simulink model "SpatialKineticsOffline"  (R2013a)
settings: Solver=ode4  StartTime=0.0  StopTime=tf  FixedStep=.001  RelTol=1e-3
PreLoadFcn:
  | load DarkLowerCoeffs
  | load DarkMiddleCoeffs
  | load DarkUpperCoeffs
  | load breaks
values from neighbouring files (symbols this model uses):
  alpha = [ -2.61*pcm -0.53*pcm ]    [SpatialKineticsOpenSourceMain.m]
  breaks = DarkLowerBreaks    [SpatialKineticsOpenSourceMain.m]
  BRIO = 4.266e7    (= 42660000)    [SpatialKineticsOpenSourceMain.m]
  cpc = 2414    [SpatialKineticsOpenSourceMain.m]
  cpp = 2414    [SpatialKineticsOpenSourceMain.m]
  DarkLowerCoeffs = ppDarkLower.coefs    [SpatialKineticsOpenSourceMain.m]
  DarkMiddleCoeffs = ppDarkMiddle.coefs    [SpatialKineticsOpenSourceMain.m]
  DarkRodWorthInserted = -5*Beta    (= -0.00815)    [SpatialKineticsOpenSourceMain.m]
  DarkUpperCoeffs = ppDarkUpper.coefs    [SpatialKineticsOpenSourceMain.m]
  downcomerTimeConstant = 5    [SpatialKineticsOpenSourceMain.m]
  downIO = 216.6*ones(1,3)    [SpatialKineticsOpenSourceMain.m]
  Kc1 = 1/(rho_secondary*V_secondary)    (= 0.00032726218348)    [SpatialKineticsOpenSourceMain.m]
  Kc2 = (h_secondary*A)/(cps*rho_secondary*V_secondary)    (= 1.23242359038)    [SpatialKineticsOpenSourceMain.m]
  Kh1 = 1/(rho_primary*V_primary)    (= 0.000447917898441)    [SpatialKineticsOpenSourceMain.m]
  Kh2 = (h_primary*A)/(cpp*rho_primary*V_primary)    (= 1.29038206968)    [SpatialKineticsOpenSourceMain.m]
  Kw1 = h_primary    (= 23800)    [SpatialKineticsOpenSourceMain.m]
  Kw2 = h_secondary    (= 24500)    [SpatialKineticsOpenSourceMain.m]
  Kw3 = A/(rho_tube*cpw*V_tube)    (= 0.000122049789882)    [SpatialKineticsOpenSourceMain.m]
  PHX_IO = [649.8 637.9 643.7]    [SpatialKineticsOpenSourceMain.m]
  PHX_PI_IO = 271.8    [SpatialKineticsOpenSourceMain.m]
  rate_pct = rate/100    [SpatialKineticsOfflineMain.m]
  rcp_activatetime = 20    [SpatialKineticsOpenSourceMain.m]
  rcpt = 0.1    [SpatialKineticsOpenSourceMain.m]
  reactor_PI_IO = 0.8574    [SpatialKineticsOpenSourceMain.m]
  SVIO = zeros(1,17)    [SpatialKineticsOpenSourceMain.m]
  Ts = 0.001    [SpatialKineticsOpenSourceMain.m]
  xfc0 = -Atemp\btemp*u0    [SpatialKineticsOpenSourceMain.m]
  zone1_IO = [1.041 0.01764 0.04848]    [SpatialKineticsOpenSourceMain.m]
  zone1_thermal_IO = [1044 658.3]    [SpatialKineticsOpenSourceMain.m]
  zone2_IO = [1.098 0.0186 0.05114]    [SpatialKineticsOpenSourceMain.m]
  zone2_thermal_IO = [1083 675.9]    [SpatialKineticsOpenSourceMain.m]
  zone3_IO = [0.9147 0.01549 0.04259]    [SpatialKineticsOpenSourceMain.m]
  zone3_thermal_IO = [1031 692.5]    [SpatialKineticsOpenSourceMain.m]
libraries: simulink x36
(part 1 of 5)
settings Model: BufferReuse=off  Creator=LabUser  LastModifiedBy=LabUser
settings DataIOCC: LimitDataPoints=off
settings OptimizationCC: BlockReduction=off  OptimizeBlockIOStorage=off  BufferReuse=off  ExpressionFolding=off  LocalBlockOutputs=off
settings HardwareCC: ProdIntDivRoundTo=Zero  ProdEndianess=LittleEndian  ProdHWDeviceType=Generic->32-bit x86 compatible
settings RTWCC: SystemTargetFile=xpctarget.tlc  TemplateMakefile=xpc_default_tmf  Description=xPC Target  ProcessScript=xpctarget_make_rtw_hook  RTWCompilerOptimization=On
settings TargetCC: CodeReplacementLibrary=XPC_BLAS  IsPILTarget=off  ParMdlRefBuildCompliant=on  ConcurrentExecutionCompliant=on  MatFileLogging=on  EnableShiftOperators=on  MATLABClassNameForMDSCustomization=xpcAperiodicCustomization

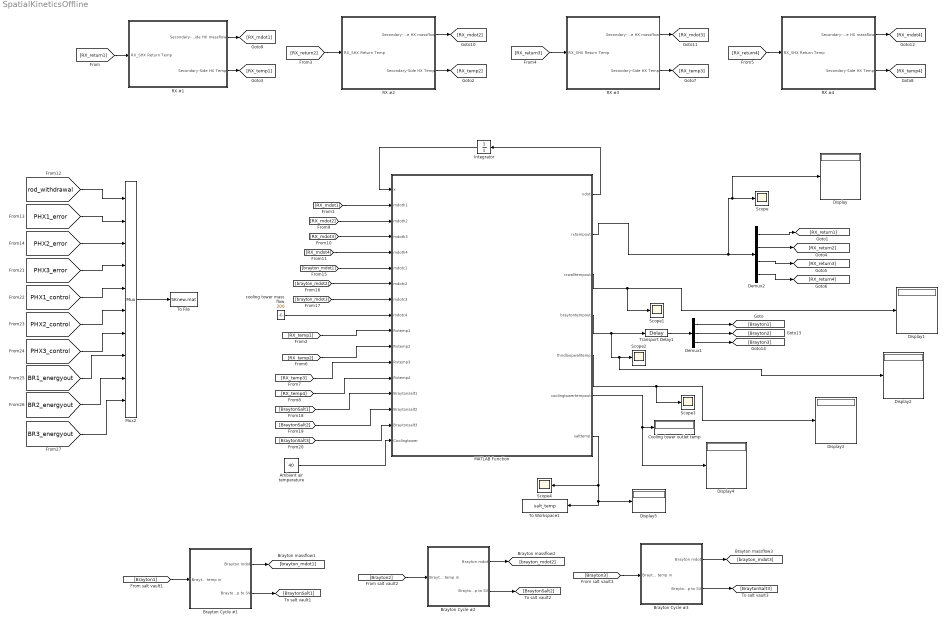
== system SpatialKineticsOffline ==
  Ambient air temperature : Constant  Value=40
  Brayton Cycle #1 : Subsystem
  Brayton Cycle #2 : Subsystem
  Brayton Cycle #3 : Subsystem
  Cooling tower outlet temp : Display
  Demux1 : Demux  Outputs=3
  Demux2 : Demux
  Display{,1..5} (6 alike) : Display
  Integrator : Integrator  InitialCondition=SVIO
  MATLAB Function : MATLAB Function  TreatAsAtomicUnit=on
  Mux2 : Mux  Inputs=10
  RX #1 : Subsystem
  RX #2 : Subsystem
  RX #3 : Subsystem
  RX #4 : Subsystem
  Scope{,1..4} (5 alike) : Scope
      Scope settings: TimeRange=100  YMin=0  YMax=85
      Scope1 settings: TimeRange=100  YMin=0  YMax=85  SaveName=ScopeData3
      Scope2 settings: TimeRange=100  YMin=0  YMax=85  SaveName=ScopeData4
      Scope3 settings: TimeRange=100  YMin=0  YMax=85  SaveName=ScopeData5
      Scope4 settings: TimeRange=100  YMin=0  YMax=85  SaveName=ScopeData6
  To File : ToFile  Filename=SKnew.mat  MatrixName=SKnew
  To Workspace1 : ToWorkspace  VariableName=salt_temp  SampleTime=-1
  Transport Delay1 : TransportDelay
  cooling tower mass flow : Constant  Value=200
  wires:
  RX #1/2(Secondary-Side HX Temp) -> [RX_temp1]
  RX #2/2(Secondary-Side HX Temp) -> [RX_temp2]
  RX #3/2(Secondary-Side HX Temp) -> [RX_temp3]
  RX #4/2(Secondary-Side HX Temp) -> [RX_temp4]
  RX #1/1(Secondary-Side HX massflow) -> [RX_mdot1]
  RX #2/1(Secondary-Side HX massflow) -> [RX_mdot2]
  RX #3/1(Secondary-Side HX massflow) -> [RX_mdot3]
  RX #4/1(Secondary-Side HX massflow) -> [RX_mdot4]
  [RX_return1] -> RX #1/1(RX_SHX Return Temp)
  [RX_return2] -> RX #2/1(RX_SHX Return Temp)
  [RX_return3] -> RX #3/1(RX_SHX Return Temp)
  [RX_return4] -> RX #4/1(RX_SHX Return Temp)
  [Brayton3] -> Brayton Cycle #3/1(Brayton temp in)
  Brayton Cycle #3/1(Brayton mdot) -> [brayton_mdot3]
  Brayton Cycle #3/2(Brayton Temp to SV) -> [BraytonSalt3]
  [Brayton1] -> Brayton Cycle #1/1(Brayton temp in)
  Brayton Cycle #1/1(Brayton mdot) -> [brayton_mdot1]
  Brayton Cycle #1/2(Brayton Temp to SV) -> [BraytonSalt1]
  [Brayton2] -> Brayton Cycle #2/1(Brayton temp in)
  Brayton Cycle #2/1(Brayton mdot) -> [brayton_mdot2]
  Brayton Cycle #2/2(Brayton Temp to SV) -> [BraytonSalt2]
  [rod_withdrawal] -> Mux2/1
  [PHX1_error] -> Mux2/2
  [PHX2_error] -> Mux2/3
  [PHX3_error] -> Mux2/4
  [PHX1_control] -> Mux2/5
  [PHX2_control] -> Mux2/6
  [PHX3_control] -> Mux2/7
  [BR1_energyout] -> Mux2/8
  [BR2_energyout] -> Mux2/9
  [BR3_energyout] -> Mux2/10
  Mux2/1 -> To File/1
  MATLAB Function/1(xdot) -> Integrator/1
  Integrator/1 -> MATLAB Function/1(x)
  MATLAB Function/2(rxtempout) -> Display/1, Scope/1, Demux2/1
  MATLAB Function/6(coolingtowertempout) -> Cooling tower outlet temp/1, Display4/1
  Transport Delay1/1 -> Demux1/1
  Demux1/1 -> [Brayton1]
  Demux1/2 -> [Brayton2]
  cooling tower mass flow/1 -> MATLAB Function/9(mdotc4)
  [brayton_mdot3] -> MATLAB Function/8(mdotc3)
  [brayton_mdot2] -> MATLAB Function/7(mdotc2)
  [brayton_mdot1] -> MATLAB Function/6(mdotc1)
  [RX_mdot4] -> MATLAB Function/5(mdoth4)
  [RX_mdot3] -> MATLAB Function/4(mdoth3)
  [RX_mdot2] -> MATLAB Function/3(mdoth2)
  [RX_mdot1] -> MATLAB Function/2(mdoth1)
  Demux2/2 -> [RX_return2]
  Demux2/3 -> [RX_return3]
  Demux2/4 -> [RX_return4]
  Demux2/1 -> [RX_return1]
  Demux1/3 -> [Brayton3]
  MATLAB Function/4(braytontempout) -> Display2/1, Scope2/1, Transport Delay1/1
  [RX_temp1] -> MATLAB Function/10(Rxtemp1)
  [RX_temp2] -> MATLAB Function/11(Rxtemp2)
  [RX_temp3] -> MATLAB Function/12(Rxtemp3)
  [RX_temp4] -> MATLAB Function/13(Rxtemp4)
  [BraytonSalt1] -> MATLAB Function/14(Braytonsalt1)
  [BraytonSalt2] -> MATLAB Function/15(Braytonsalt2)
  [BraytonSalt3] -> MATLAB Function/16(Braytonsalt3)
  Ambient air temperature/1 -> MATLAB Function/17(Coolingtower)
  MATLAB Function/3(rxwalltempout) -> Scope1/1, Display1/1
  MATLAB Function/5(thirdloopwalltemp) -> Scope3/1, Display3/1
  MATLAB Function/7(salttemp) -> To Workspace1/1, Display5/1, Scope4/1

== system SpatialKineticsOffline/Brayton Cycle #1 ==
  Brayton temp in : Inport
  Brayton Cycle Parameters : FromWorkspace  VariableName=[0,eta_C,eta_T,r,cpCO2Turbine,cpCO2Compressor,rhoCO2,tau_t]  SampleTime=0
  Compressor Inlet Temp : Constant  Value=10
  Display : Display
  Electricity Extraction : Display
  Generator Efficiency : Gain  Gain=0.60
  Integrator : Integrator  InitialCondition=BRIO
  MATLAB Function : MATLAB Function  TreatAsAtomicUnit=on
  Mux4 : Mux  Inputs=2
  Terminator : Terminator
  Watts to MW : Gain  Gain=1/1000000
  kg/s : Constant  Value=500
  Brayton mdot : Outport
  Brayton Temp to SV : Outport  Port=2
  tag scope: BR1_energyout=global
  wires:
  Brayton Cycle Parameters/1 -> MATLAB Function/4(constants)
  Integrator/1 -> MATLAB Function/5(x), Display/1
  kg/s/1 -> MATLAB Function/3(mdot), Brayton mdot/1
  MATLAB Function/4(xdot) -> Integrator/1
  Brayton temp in/1 -> MATLAB Function/2(Tturb_in)
  Compressor Inlet Temp/1 -> MATLAB Function/1(Tcomp_in)
  Generator Efficiency/1 -> [BR1_energyout], Electricity Extraction/1
  Mux4/1 -> Terminator/1
  MATLAB Function/3(Tcomp_out) -> Brayton Temp to SV/1, Mux4/2
  MATLAB Function/1(y) -> Watts to MW/1
  Watts to MW/1 -> Generator Efficiency/1
  MATLAB Function/2(Tturb_out) -> Mux4/1

== system SpatialKineticsOffline/Brayton Cycle #2 ==
  Brayton temp in : Inport
  Brayton Cycle Parameters2 : FromWorkspace  VariableName=[0,eta_C,eta_T,r,cpCO2Turbine,cpCO2Compressor,rhoCO2,tau_t]  SampleTime=0
  Compressor Inlet Temp2 : Constant  Value=10
  Display : Display
  Electricity Extraction2 : Display
  Generator Efficiency2 : Gain  Gain=0.60
  Integrator3 : Integrator  InitialCondition=BRIO
  MATLAB Function4 : MATLAB Function  TreatAsAtomicUnit=on
  Mechanical Power Extraction2 : Display
  Mux4 : Mux  Inputs=2
  Terminator : Terminator
  Watts to MW3 : Gain  Gain=1/1000000
  kg/s2 : Constant  Value=500
  Brayton mdot : Outport
  Brayton Temp to SV : Outport  Port=2
  tag scope: BR2_energyout=global
  wires:
  Brayton Cycle Parameters2/1 -> MATLAB Function4/4(constants)
  Integrator3/1 -> MATLAB Function4/5(x), Display/1
  kg/s2/1 -> MATLAB Function4/3(mdot), Brayton mdot/1
  MATLAB Function4/4(xdot) -> Integrator3/1
  Brayton temp in/1 -> MATLAB Function4/2(Tturb_in)
  Compressor Inlet Temp2/1 -> MATLAB Function4/1(Tcomp_in)
  Generator Efficiency2/1 -> [BR2_energyout], Electricity Extraction2/1
  Mux4/1 -> Terminator/1
  MATLAB Function4/3(Tcomp_out) -> Brayton Temp to SV/1, Mux4/2
  MATLAB Function4/1(y) -> Watts to MW3/1
  Watts to MW3/1 -> Generator Efficiency2/1, Mechanical Power Extraction2/1
  MATLAB Function4/2(Tturb_out) -> Mux4/1

== system SpatialKineticsOffline/Brayton Cycle #3 ==
  Brayton temp in : Inport
  Brayton Cycle Parameters2 : FromWorkspace  VariableName=[0,eta_C,eta_T,r,cpCO2Turbine,cpCO2Compressor,rhoCO2,tau_t]  SampleTime=0
  Compressor Inlet Temp2 : Constant  Value=10
  Display : Display
  Electricity Extraction2 : Display
  Generator Efficiency2 : Gain  Gain=0.60
  Integrator3 : Integrator  InitialCondition=BRIO
  MATLAB Function4 : MATLAB Function  TreatAsAtomicUnit=on
  Mechanical Power Extraction2 : Display
  Mux4 : Mux  Inputs=2
  Terminator : Terminator
  Watts to MW3 : Gain  Gain=1/1000000
  kg/s2 : Constant  Value=500
  Brayton mdot : Outport
  Brayton Temp to SV : Outport  Port=2
  tag scope: BR3_energyout=global
  wires:
  Brayton Cycle Parameters2/1 -> MATLAB Function4/4(constants)
  Integrator3/1 -> Display/1, MATLAB Function4/5(x)
  kg/s2/1 -> MATLAB Function4/3(mdot), Brayton mdot/1
  MATLAB Function4/4(xdot) -> Integrator3/1
  Brayton temp in/1 -> MATLAB Function4/2(Tturb_in)
  Compressor Inlet Temp2/1 -> MATLAB Function4/1(Tcomp_in)
  Generator Efficiency2/1 -> [BR3_energyout], Electricity Extraction2/1
  Mux4/1 -> Terminator/1
  MATLAB Function4/3(Tcomp_out) -> Brayton Temp to SV/1, Mux4/2
  MATLAB Function4/1(y) -> Watts to MW3/1
  Watts to MW3/1 -> Generator Efficiency2/1, Mechanical Power Extraction2/1
  MATLAB Function4/2(Tturb_out) -> Mux4/1

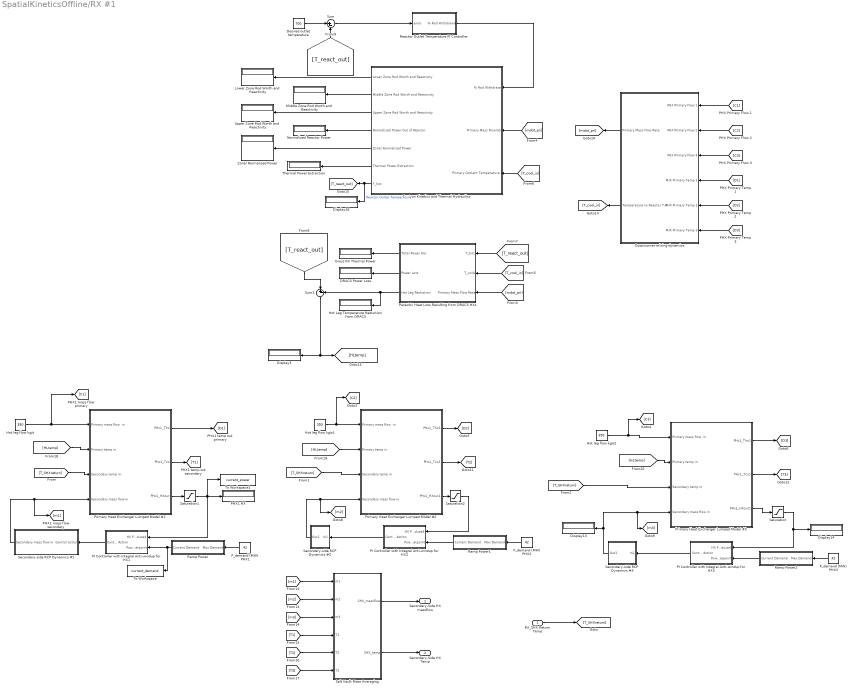
== system SpatialKineticsOffline/RX #1 ==
  RX_SHX Return Temp : Inport
  DRACS Power Loss : Display
  Desired outlet temperature : Constant  Value=700
  Display{3,13..14,16} (4 alike) : Display
  Downcomer mixing dynamics : Subsystem
  Gross RX Thermal Power : Display
  Hot Leg Temperature Reduction from DRACS : Display
  Hot leg flow kg/s : Constant  Value=350
  Hot leg flow kg/s1 : Constant  Value=350
  Hot leg flow kg/s2 : Constant  Value=350
  Lower Zone Rod Worth and Reactivity : Display
  Middle Zone Rod Worth and Reactivity : Display
  Neutron Kinetics and Thermal Hydraulics : Subsystem
  Normalized Reactor Power : Display
  PHX1 HX : Display
  PI Controller with Integral Anti-windup for HX1 : Subsystem
  PI Controller with Integral Anti-windup for HX2 : Subsystem
  PI Controller with Integral Anti-windup for HX3 : Subsystem
  P_demand (MW) PHX1 : Constant  Value=42
  P_demand (MW) PHX2 : Constant  Value=42
  P_demand (MW) PHX3 : Constant  Value=42
  Parasitic Heat Loss Resulting from DRACS HXs : Subsystem
  Primary Heat Exchanger Lumped Model #1 : Subsystem
  Primary Heat Exchanger Lumped Model #2 : Subsystem
  Primary Heat Exchanger Lumped Model #3 : Subsystem
  Ramp Power : Subsystem
  Ramp Power1 : Subsystem
  Ramp Power2 : Subsystem
  Reactor Outlet Temperature PI Controller : Subsystem
  Salt Vault Mass Averaging : MATLAB Function  TreatAsAtomicUnit=on
  Saturation : Saturate  UpperLimit=inf  LowerLimit=0
  Saturation1 : Saturate  UpperLimit=inf  LowerLimit=0
  Saturation2 : Saturate  UpperLimit=inf  LowerLimit=0
  Secondary-side RCP Dynamics #1 : Subsystem
  Secondary-side RCP Dynamics #2 : Subsystem
  Secondary-side RCP Dynamics #3 : Subsystem
  Sum : Sum  Inputs=|+-
  Sum3 : Sum  Inputs=|+-
  Thermal Power Extraction : Display
  To Workspace : ToWorkspace  VariableName=current_demand  SampleTime=-1
  To Workspace1 : ToWorkspace  VariableName=current_power  SampleTime=-1
  Upper Zone Rod Worth and Reactivity : Display
  Zonal Normalized Power : Display
  Secondary-Side HX massflow : Outport
  Secondary-Side HX Temp : Outport  Port=2
  wires:
  Reactor Outlet Temperature PI Controller/1(% Rod Withdrawn) -> Neutron Kinetics and Thermal Hydraulics/1(% Rod Withdrawn)
  Parasitic Heat Loss Resulting from DRACS HXs/3(Hot Leg Reduction) -> Hot Leg Temperature Reduction from DRACS/1, Sum3/2
  Parasitic Heat Loss Resulting from DRACS HXs/1(Total Power Out) -> Gross RX Thermal Power/1
  Parasitic Heat Loss Resulting from DRACS HXs/2(Power Lost) -> DRACS Power Loss/1
  Sum3/1 -> Display3/1, [HLtemp]
  [C1] -> Downcomer mixing dynamics/1(PHX Primary Flow 1)
  [C2] -> Downcomer mixing dynamics/2(PHX Primary Flow 2)
  [C3] -> Downcomer mixing dynamics/3(PHX Primary Flow 3)
  [D1] -> Downcomer mixing dynamics/4(PHX Primary Temp 1)
  [D2] -> Downcomer mixing dynamics/5(PHX Primary Temp 2)
  [D3] -> Downcomer mixing dynamics/6(PHX Primary Temp 3)
  [m1] -> Salt Vault Mass Averaging/1(m1)
  [m2] -> Salt Vault Mass Averaging/2(m2)
  [m3] -> Salt Vault Mass Averaging/3(m3)
  [T1] -> Salt Vault Mass Averaging/4(T1)
  [T2] -> Salt Vault Mass Averaging/5(T2)
  [T3] -> Salt Vault Mass Averaging/6(T3)
  Neutron Kinetics and Thermal Hydraulics/6(Thermal Power Extraction) -> Thermal Power Extraction/1
  Neutron Kinetics and Thermal Hydraulics/5(Zonal Normalized Power) -> Zonal Normalized Power/1
  Neutron Kinetics and Thermal Hydraulics/4(Normalized Power Out of Reactor) -> Normalized Reactor Power/1
  Neutron Kinetics and Thermal Hydraulics/1(Lower Zone Rod Worth and Reactivity) -> Lower Zone Rod Worth and Reactivity/1
  Neutron Kinetics and Thermal Hydraulics/2(Middle Zone Rod Worth and Reactivity) -> Middle Zone Rod Worth and Reactivity/1
  Neutron Kinetics and Thermal Hydraulics/3(Upper Zone Rod Worth and Reactivity) -> Upper Zone Rod Worth and Reactivity/1
  Sum/1 -> Reactor Outlet Temperature PI Controller/1(error)
  Desired outlet temperature/1 -> Sum/1
  Salt Vault Mass Averaging/2(SHX_temp) -> Secondary-Side HX Temp/1
  Salt Vault Mass Averaging/1(SHX_massflow) -> Secondary-Side HX massflow/1
  RX_SHX Return Temp/1 -> [T_SHXreturn]
  Hot leg flow kg/s/1 -> [C1], Primary Heat Exchanger Lumped Model #1/1(Primary mass flow  in)
  [HLtemp] -> Primary Heat Exchanger Lumped Model #1/2(Primary temp in)
  Saturation1/1 -> To Workspace1/1, PI Controller with Integral Anti-windup for HX1/1(HX Power Produced), PHX1 HX/1
  PI Controller with Integral Anti-windup for HX1/1(Control Action) -> Secondary-side RCP Dynamics #1/1(Control action)
  Secondary-side RCP Dynamics #1/1(Secondary mass flow in) -> [m1], Primary Heat Exchanger Lumped Model #1/4(Secondary mass flow in)
  [T_SHXreturn] -> Primary Heat Exchanger Lumped Model #1/3(Secondary temp in)
  Primary Heat Exchanger Lumped Model #1/1(PHx1_Tho) -> [D1]
  Primary Heat Exchanger Lumped Model #1/2(PHx1_Tco) -> [T1]
  Primary Heat Exchanger Lumped Model #1/3(PHx1_HXout) -> Saturation1/1
  Hot leg flow kg/s1/1 -> [C2], Primary Heat Exchanger Lumped Model #2/1(Primary mass flow  in)
  Primary Heat Exchanger Lumped Model #2/3(PHx1_HXout1) -> Saturation2/1
  [HLtemp] -> Primary Heat Exchanger Lumped Model #2/2(Primary temp in)
  PI Controller with Integral Anti-windup for HX2/1(Control Action) -> Secondary-side RCP Dynamics #2/1(In1)
  Secondary-side RCP Dynamics #2/1(Out1) -> [m2], Primary Heat Exchanger Lumped Model #2/4(Secondary mass flow in)
  Saturation2/1 -> PI Controller with Integral Anti-windup for HX2/1(HX Power Produced)
  [T_SHXreturn] -> Primary Heat Exchanger Lumped Model #2/3(Secondary temp in)
  Primary Heat Exchanger Lumped Model #2/1(PHx1_Tho1) -> [D2]
  Primary Heat Exchanger Lumped Model #2/2(PHx1_Tco1) -> [T2]
  Hot leg flow kg/s2/1 -> [C3], Primary Heat Exchanger Lumped Model #3/1(Primary mass flow  in)
  Saturation/1 -> PI Controller with Integral Anti-windup for HX3/1(HX Power Produced), Display14/1
  PI Controller with Integral Anti-windup for HX3/1(Control Action) -> Secondary-side RCP Dynamics #3/1(In1)
  Secondary-side RCP Dynamics #3/1(Out1) -> [m3], Primary Heat Exchanger Lumped Model #3/4(Secondary mass flow in), Display13/1
  [HLtemp] -> Primary Heat Exchanger Lumped Model #3/2(Primary temp in)
  [T_SHXreturn] -> Primary Heat Exchanger Lumped Model #3/3(Secondary temp in)
  Primary Heat Exchanger Lumped Model #3/2(PHx1_Tco1) -> [T3]
  Primary Heat Exchanger Lumped Model #3/1(PHx1_Tho1) -> [D3]
  Primary Heat Exchanger Lumped Model #3/3(PHx1_HXout1) -> Saturation/1
  Downcomer mixing dynamics/1(Primary Mass Flow Rate) -> [mdot_pri]
  [mdot_pri] -> Parasitic Heat Loss Resulting from DRACS HXs/3(Primary Mass Flow Rate)
  [mdot_pri] -> Neutron Kinetics and Thermal Hydraulics/2(Primary Mass Flowrate)
  Downcomer mixing dynamics/2(Temperature to Reactor T-H) -> [T_cool_in]
  [T_cool_in] -> Parasitic Heat Loss Resulting from DRACS HXs/2(T_cold)
  [T_cool_in] -> Neutron Kinetics and Thermal Hydraulics/3(Primary Coolant Temperature In)
  Neutron Kinetics and Thermal Hydraulics/7(T_hot) -> Display16/1, [T_react_out]  "Reactor Outlet Temperature"
  [T_react_out] -> Parasitic Heat Loss Resulting from DRACS HXs/1("T_hot ")
  [T_react_out] -> Sum3/1
  [T_react_out] -> Sum/2
  Ramp Power/1(Current Demand) -> PI Controller with Integral Anti-windup for HX1/2(Power Setpoint), To Workspace/1
  P_demand (MW) PHX1/1 -> Ramp Power/1(Max Demand)
  Ramp Power1/1(Current Demand) -> PI Controller with Integral Anti-windup for HX2/2(Power Setpoint)
  P_demand (MW) PHX2/1 -> Ramp Power1/1(Max Demand)
  Ramp Power2/1(Current Demand) -> PI Controller with Integral Anti-windup for HX3/2(Power Setpoint)
  P_demand (MW) PHX3/1 -> Ramp Power2/1(Max Demand)

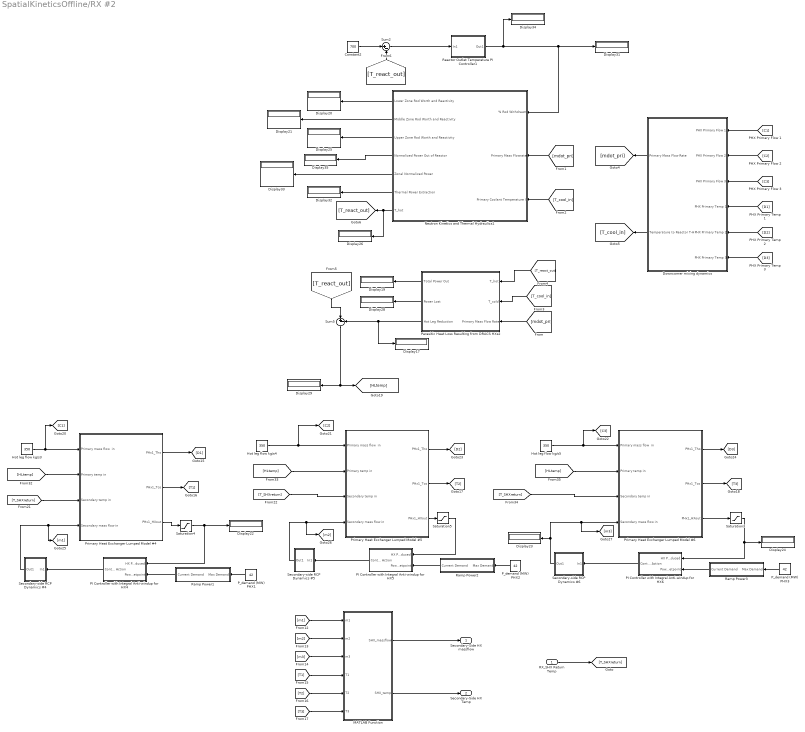
== system SpatialKineticsOffline/RX #2 ==
  RX_SHX Return Temp : Inport
  Constant2 : Constant  Value=700
  Display{17,19..26,28..29,31..35} (16 alike) : Display
  Downcomer mixing dynamics : Subsystem
  Hot leg flow kg/s3 : Constant  Value=350
  Hot leg flow kg/s4 : Constant  Value=350
  Hot leg flow kg/s5 : Constant  Value=350
  MATLAB Function : MATLAB Function  TreatAsAtomicUnit=on
  Neutron Kinetics and Thermal Hydraulics1 : Subsystem
  PI Controller with Integral Anti-windup for HX4 : Subsystem
  PI Controller with Integral Anti-windup for HX5 : Subsystem
  PI Controller with Integral Anti-windup for HX6 : Subsystem
  P_demand (MW) PHX1 : Constant  Value=42
  P_demand (MW) PHX2 : Constant  Value=42
  P_demand (MW) PHX3 : Constant  Value=42
  Parasitic Heat Loss Resulting from DRACS HXs2 : Subsystem
  Primary Heat Exchanger Lumped Model #4 : Subsystem
  Primary Heat Exchanger Lumped Model #5 : Subsystem
  Primary Heat Exchanger Lumped Model #6 : Subsystem
  Ramp Power1 : Subsystem
  Ramp Power2 : Subsystem
  Ramp Power3 : Subsystem
  Reactor Outlet Temperature PI Controller1 : Subsystem
  Saturation3 : Saturate  UpperLimit=inf  LowerLimit=0
  Saturation4 : Saturate  UpperLimit=inf  LowerLimit=0
  Saturation5 : Saturate  UpperLimit=inf  LowerLimit=0
  Secondary-side RCP Dynamics #4 : Subsystem
  Secondary-side RCP Dynamics #5 : Subsystem
  Secondary-side RCP Dynamics #6 : Subsystem
  Sum2 : Sum  Inputs=|+-
  Sum5 : Sum  Inputs=|+-
  Secondary-Side HX massflow : Outport
  Secondary-Side HX Temp : Outport  Port=2
  wires:
  Reactor Outlet Temperature PI Controller1/1(Out1) -> Neutron Kinetics and Thermal Hydraulics1/1(% Rod Withdrawn), Display31/1, Display34/1
  Parasitic Heat Loss Resulting from DRACS HXs2/3(Hot Leg Reduction) -> Sum5/2, Display17/1
  Parasitic Heat Loss Resulting from DRACS HXs2/1(Total Power Out) -> Display19/1
  Parasitic Heat Loss Resulting from DRACS HXs2/2(Power Lost) -> Display28/1
  Sum5/1 -> Display29/1, [HLtemp]
  Neutron Kinetics and Thermal Hydraulics1/6(Thermal Power Extraction) -> Display32/1
  Neutron Kinetics and Thermal Hydraulics1/5(Zonal Normalized Power) -> Display33/1
  Neutron Kinetics and Thermal Hydraulics1/4(Normalized Power Out of Reactor) -> Display35/1
  Neutron Kinetics and Thermal Hydraulics1/1(Lower Zone Rod Worth and Reactivity) -> Display20/1
  Neutron Kinetics and Thermal Hydraulics1/2(Middle Zone Rod Worth and Reactivity) -> Display21/1
  Neutron Kinetics and Thermal Hydraulics1/3(Upper Zone Rod Worth and Reactivity) -> Display25/1
  Sum2/1 -> Reactor Outlet Temperature PI Controller1/1(In1)
  Constant2/1 -> Sum2/1
  [m1] -> MATLAB Function/1(m1)
  [m2] -> MATLAB Function/2(m2)
  [m3] -> MATLAB Function/3(m3)
  [T1] -> MATLAB Function/4(T1)
  [T2] -> MATLAB Function/5(T2)
  [T3] -> MATLAB Function/6(T3)
  MATLAB Function/2(SHX_temp) -> Secondary-Side HX Temp/1
  MATLAB Function/1(SHX_massflow) -> Secondary-Side HX massflow/1
  RX_SHX Return Temp/1 -> [T_SHXreturn]
  [C1] -> Downcomer mixing dynamics/1(PHX Primary Flow 1)
  [C2] -> Downcomer mixing dynamics/2(PHX Primary Flow 2)
  [C3] -> Downcomer mixing dynamics/3(PHX Primary Flow 3)
  [D1] -> Downcomer mixing dynamics/4(PHX Primary Temp 1)
  [D2] -> Downcomer mixing dynamics/5(PHX Primary Temp 2)
  [D3] -> Downcomer mixing dynamics/6(PHX Primary Temp 3)
  Hot leg flow kg/s3/1 -> [C1], Primary Heat Exchanger Lumped Model #4/1(Primary mass flow  in)
  Hot leg flow kg/s4/1 -> [C2], Primary Heat Exchanger Lumped Model #5/1(Primary mass flow  in)
  Hot leg flow kg/s5/1 -> [C3], Primary Heat Exchanger Lumped Model #6/1(Primary mass flow  in)
  Primary Heat Exchanger Lumped Model #5/3(PHx1_HXout) -> Saturation5/1
  [HLtemp] -> Primary Heat Exchanger Lumped Model #4/2(Primary temp in)
  [HLtemp] -> Primary Heat Exchanger Lumped Model #5/2(Primary temp in)
  [HLtemp] -> Primary Heat Exchanger Lumped Model #6/2(Primary temp in)
  Saturation3/1 -> PI Controller with Integral Anti-windup for HX6/1(HX Power Produced), Display24/1
  Saturation4/1 -> PI Controller with Integral Anti-windup for HX4/1(HX Power Produced), Display22/1
  Ramp Power1/1(Current Demand) -> PI Controller with Integral Anti-windup for HX4/2(Power Setpoint)
  Ramp Power2/1(Current Demand) -> PI Controller with Integral Anti-windup for HX5/2(Power Setpoint)
  Ramp Power3/1(Current Demand) -> PI Controller with Integral Anti-windup for HX6/2(Power Setpoint)
  PI Controller with Integral Anti-windup for HX4/1(Control Action) -> Secondary-side RCP Dynamics #4/1(In1)
  PI Controller with Integral Anti-windup for HX5/1(Control Action) -> Secondary-side RCP Dynamics #5/1(In1)
  Secondary-side RCP Dynamics #5/1(Out1) -> [m2], Primary Heat Exchanger Lumped Model #5/4(Secondary mass flow in)
  PI Controller with Integral Anti-windup for HX6/1(Control Action) -> Secondary-side RCP Dynamics #6/1(In1)
  Saturation5/1 -> PI Controller with Integral Anti-windup for HX5/1(HX Power Produced)
  [T_SHXreturn] -> Primary Heat Exchanger Lumped Model #4/3(Secondary temp in)
  [T_SHXreturn] -> Primary Heat Exchanger Lumped Model #5/3(Secondary temp in)
  [T_SHXreturn] -> Primary Heat Exchanger Lumped Model #6/3(Secondary temp in)
  Primary Heat Exchanger Lumped Model #4/3(PHx1_HXout) -> Saturation4/1
  Secondary-side RCP Dynamics #4/1(Out1) -> [m1], Primary Heat Exchanger Lumped Model #4/4(Secondary mass flow in)
  Primary Heat Exchanger Lumped Model #4/1(PHx1_Tho) -> [D1]
  Primary Heat Exchanger Lumped Model #4/2(PHx1_Tco) -> [T1]
  Primary Heat Exchanger Lumped Model #5/2(PHx1_Tco) -> [T2]
  Primary Heat Exchanger Lumped Model #5/1(PHx1_Tho) -> [D2]
  Secondary-side RCP Dynamics #6/1(Out1) -> [m3], Primary Heat Exchanger Lumped Model #6/4(Secondary mass flow in), Display23/1
  Primary Heat Exchanger Lumped Model #6/3(PHx1_HXout) -> Saturation3/1
  Primary Heat Exchanger Lumped Model #6/2(PHx1_Tco) -> [T3]
  Primary Heat Exchanger Lumped Model #6/1(PHx1_Tho) -> [D3]
  Downcomer mixing dynamics/1(Primary Mass Flow Rate) -> [mdot_pri]
  [mdot_pri] -> Parasitic Heat Loss Resulting from DRACS HXs2/3(Primary Mass Flow Rate)
  [mdot_pri] -> Neutron Kinetics and Thermal Hydraulics1/2(Primary Mass Flowrate)
  Downcomer mixing dynamics/2(Temperature to Reactor T-H) -> [T_cool_in]
  [T_cool_in] -> Neutron Kinetics and Thermal Hydraulics1/3(Primary Coolant Temperature In)
  [T_cool_in] -> Parasitic Heat Loss Resulting from DRACS HXs2/2(T_cold)
  Neutron Kinetics and Thermal Hydraulics1/7(T_hot) -> Display26/1, [T_react_out]
  [T_react_out] -> Parasitic Heat Loss Resulting from DRACS HXs2/1("T_hot ")
  [T_react_out] -> Sum5/1
  [T_react_out] -> Sum2/2
  P_demand (MW) PHX1/1 -> Ramp Power1/1(Max Demand)
  P_demand (MW) PHX2/1 -> Ramp Power2/1(Max Demand)
  P_demand (MW) PHX3/1 -> Ramp Power3/1(Max Demand)

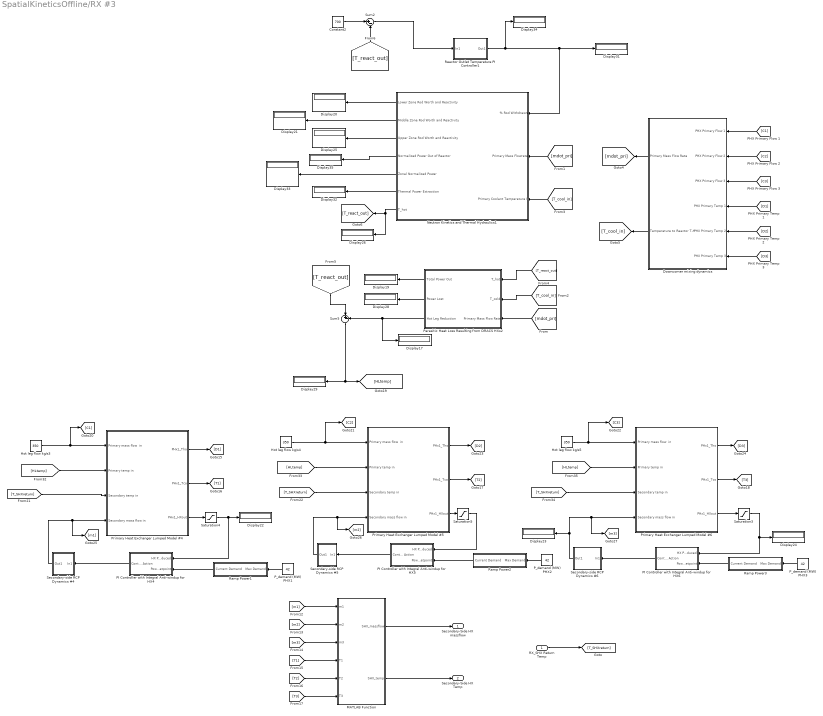
== system SpatialKineticsOffline/RX #3 ==
  RX_SHX Return Temp : Inport
  Constant2 : Constant  Value=700
  Display{17,19..26,28..29,31..35} (16 alike) : Display
  Downcomer mixing dynamics : Subsystem
  Hot leg flow kg/s3 : Constant  Value=350
  Hot leg flow kg/s4 : Constant  Value=350
  Hot leg flow kg/s5 : Constant  Value=350
  MATLAB Function : MATLAB Function  TreatAsAtomicUnit=on
  Neutron Kinetics and Thermal Hydraulics1 : Subsystem
  PI Controller with Integral Anti-windup for HX4 : Subsystem
  PI Controller with Integral Anti-windup for HX5 : Subsystem
  PI Controller with Integral Anti-windup for HX6 : Subsystem
  P_demand (MW) PHX1 : Constant  Value=42
  P_demand (MW) PHX2 : Constant  Value=42
  P_demand (MW) PHX3 : Constant  Value=42
  Parasitic Heat Loss Resulting from DRACS HXs2 : Subsystem
  Primary Heat Exchanger Lumped Model #4 : Subsystem
  Primary Heat Exchanger Lumped Model #5 : Subsystem
  Primary Heat Exchanger Lumped Model #6 : Subsystem
  Ramp Power1 : Subsystem
  Ramp Power2 : Subsystem
  Ramp Power3 : Subsystem
  Reactor Outlet Temperature PI Controller1 : Subsystem
  Saturation3 : Saturate  UpperLimit=inf  LowerLimit=0
  Saturation4 : Saturate  UpperLimit=inf  LowerLimit=0
  Saturation5 : Saturate  UpperLimit=inf  LowerLimit=0
  Secondary-side RCP Dynamics #4 : Subsystem
  Secondary-side RCP Dynamics #5 : Subsystem
  Secondary-side RCP Dynamics #6 : Subsystem
  Sum2 : Sum  Inputs=|+-
  Sum5 : Sum  Inputs=|+-
  Secondary-Side HX massflow : Outport
  Secondary-Side HX Temp : Outport  Port=2
  wires:
  Reactor Outlet Temperature PI Controller1/1(Out1) -> Neutron Kinetics and Thermal Hydraulics1/1(% Rod Withdrawn), Display31/1, Display34/1
  Parasitic Heat Loss Resulting from DRACS HXs2/3(Hot Leg Reduction) -> Sum5/2, Display17/1
  Parasitic Heat Loss Resulting from DRACS HXs2/1(Total Power Out) -> Display19/1
  Parasitic Heat Loss Resulting from DRACS HXs2/2(Power Lost) -> Display28/1
  Sum5/1 -> Display29/1, [HLtemp]
  Neutron Kinetics and Thermal Hydraulics1/6(Thermal Power Extraction) -> Display32/1
  Neutron Kinetics and Thermal Hydraulics1/5(Zonal Normalized Power) -> Display33/1
  Neutron Kinetics and Thermal Hydraulics1/4(Normalized Power Out of Reactor) -> Display35/1
  Neutron Kinetics and Thermal Hydraulics1/1(Lower Zone Rod Worth and Reactivity) -> Display20/1
  Neutron Kinetics and Thermal Hydraulics1/2(Middle Zone Rod Worth and Reactivity) -> Display21/1
  Neutron Kinetics and Thermal Hydraulics1/3(Upper Zone Rod Worth and Reactivity) -> Display25/1
  Sum2/1 -> Reactor Outlet Temperature PI Controller1/1(In1)
  Constant2/1 -> Sum2/1
  [m1] -> MATLAB Function/1(m1)
  [m2] -> MATLAB Function/2(m2)
  [m3] -> MATLAB Function/3(m3)
  [T1] -> MATLAB Function/4(T1)
  [T2] -> MATLAB Function/5(T2)
  [T3] -> MATLAB Function/6(T3)
  MATLAB Function/2(SHX_temp) -> Secondary-Side HX Temp/1
  MATLAB Function/1(SHX_massflow) -> Secondary-Side HX massflow/1
  RX_SHX Return Temp/1 -> [T_SHXreturn]
  [C1] -> Downcomer mixing dynamics/1(PHX Primary Flow 1)
  [C2] -> Downcomer mixing dynamics/2(PHX Primary Flow 2)
  [C3] -> Downcomer mixing dynamics/3(PHX Primary Flow 3)
  [D1] -> Downcomer mixing dynamics/4(PHX Primary Temp 1)
  [D2] -> Downcomer mixing dynamics/5(PHX Primary Temp 2)
  [D3] -> Downcomer mixing dynamics/6(PHX Primary Temp 3)
  Hot leg flow kg/s3/1 -> [C1], Primary Heat Exchanger Lumped Model #4/1(Primary mass flow  in)
  Hot leg flow kg/s4/1 -> [C2], Primary Heat Exchanger Lumped Model #5/1(Primary mass flow  in)
  Hot leg flow kg/s5/1 -> [C3], Primary Heat Exchanger Lumped Model #6/1(Primary mass flow  in)
  Primary Heat Exchanger Lumped Model #5/3(PHx1_HXout) -> Saturation5/1
  [HLtemp] -> Primary Heat Exchanger Lumped Model #4/2(Primary temp in)
  [HLtemp] -> Primary Heat Exchanger Lumped Model #5/2(Primary temp in)
  [HLtemp] -> Primary Heat Exchanger Lumped Model #6/2(Primary temp in)
  Primary Heat Exchanger Lumped Model #4/3(PHx1_HXout) -> Saturation4/1
  Primary Heat Exchanger Lumped Model #6/3(PHx1_HXout) -> Saturation3/1
  Saturation3/1 -> PI Controller with Integral Anti-windup for HX6/1(HX Power Produced), Display24/1
  Saturation4/1 -> PI Controller with Integral Anti-windup for HX4/1(HX Power Produced), Display22/1
  Ramp Power1/1(Current Demand) -> PI Controller with Integral Anti-windup for HX4/2(Power Setpoint)
  Ramp Power2/1(Current Demand) -> PI Controller with Integral Anti-windup for HX5/2(Power Setpoint)
  Ramp Power3/1(Current Demand) -> PI Controller with Integral Anti-windup for HX6/2(Power Setpoint)
  PI Controller with Integral Anti-windup for HX4/1(Control Action) -> Secondary-side RCP Dynamics #4/1(In1)
  Secondary-side RCP Dynamics #4/1(Out1) -> [m1], Primary Heat Exchanger Lumped Model #4/4(Secondary mass flow in)
  PI Controller with Integral Anti-windup for HX5/1(Control Action) -> Secondary-side RCP Dynamics #5/1(In1)
  Secondary-side RCP Dynamics #5/1(Out1) -> [m2], Primary Heat Exchanger Lumped Model #5/4(Secondary mass flow in)
  PI Controller with Integral Anti-windup for HX6/1(Control Action) -> Secondary-side RCP Dynamics #6/1(In1)
  Secondary-side RCP Dynamics #6/1(Out1) -> [m3], Primary Heat Exchanger Lumped Model #6/4(Secondary mass flow in), Display23/1
  Saturation5/1 -> PI Controller with Integral Anti-windup for HX5/1(HX Power Produced)
  [T_SHXreturn] -> Primary Heat Exchanger Lumped Model #4/3(Secondary temp in)
  [T_SHXreturn] -> Primary Heat Exchanger Lumped Model #5/3(Secondary temp in)
  [T_SHXreturn] -> Primary Heat Exchanger Lumped Model #6/3(Secondary temp in)
  Primary Heat Exchanger Lumped Model #4/2(PHx1_Tco) -> [T1]
  Primary Heat Exchanger Lumped Model #4/1(PHx1_Tho) -> [D1]
  Primary Heat Exchanger Lumped Model #5/2(PHx1_Tco) -> [T2]
  Primary Heat Exchanger Lumped Model #5/1(PHx1_Tho) -> [D2]
  Primary Heat Exchanger Lumped Model #6/2(PHx1_Tco) -> [T3]
  Primary Heat Exchanger Lumped Model #6/1(PHx1_Tho) -> [D3]
  Downcomer mixing dynamics/1(Primary Mass Flow Rate) -> [mdot_pri]
  [mdot_pri] -> Parasitic Heat Loss Resulting from DRACS HXs2/3(Primary Mass Flow Rate)
  [mdot_pri] -> Neutron Kinetics and Thermal Hydraulics1/2(Primary Mass Flowrate)
  Downcomer mixing dynamics/2(Temperature to Reactor T-H) -> [T_cool_in]
  [T_cool_in] -> Parasitic Heat Loss Resulting from DRACS HXs2/2(T_cold)
  [T_cool_in] -> Neutron Kinetics and Thermal Hydraulics1/3(Primary Coolant Temperature In)
  Neutron Kinetics and Thermal Hydraulics1/7(T_hot) -> Display26/1, [T_react_out]
  [T_react_out] -> Parasitic Heat Loss Resulting from DRACS HXs2/1("T_hot ")
  [T_react_out] -> Sum5/1
  [T_react_out] -> Sum2/2
  P_demand (MW) PHX1/1 -> Ramp Power1/1(Max Demand)
  P_demand (MW) PHX2/1 -> Ramp Power2/1(Max Demand)
  P_demand (MW) PHX3/1 -> Ramp Power3/1(Max Demand)

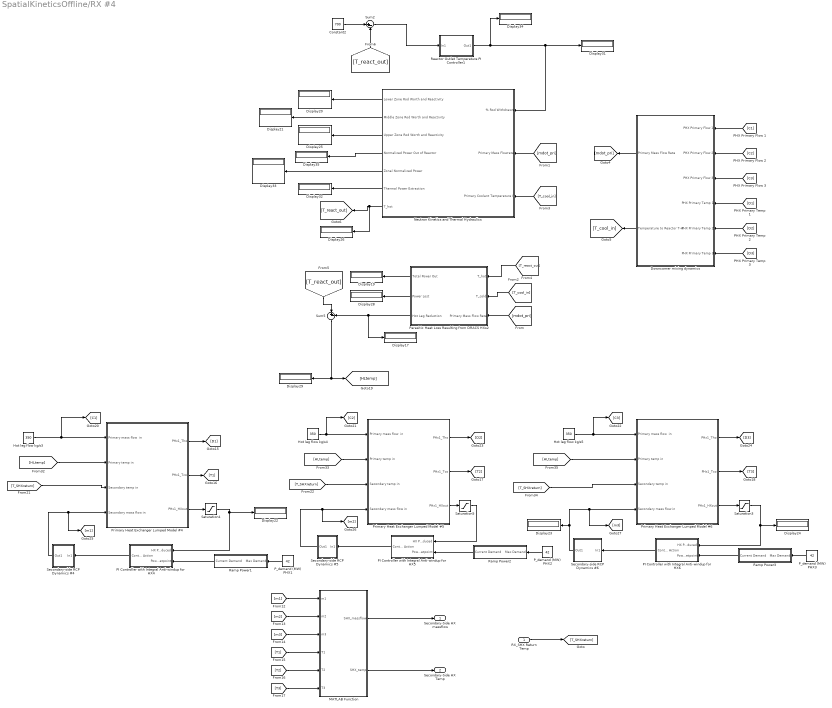
== system SpatialKineticsOffline/RX #4 ==
  RX_SHX Return Temp : Inport
  Constant2 : Constant  Value=700
  Display{17,19..26,28..29,31..35} (16 alike) : Display
  Downcomer mixing dynamics : Subsystem
  Hot leg flow kg/s3 : Constant  Value=350
  Hot leg flow kg/s4 : Constant  Value=350
  Hot leg flow kg/s5 : Constant  Value=350
  MATLAB Function : MATLAB Function  TreatAsAtomicUnit=on
  Neutron Kinetics and Thermal Hydraulics : Subsystem
  PI Controller with Integral Anti-windup for HX4 : Subsystem
  PI Controller with Integral Anti-windup for HX5 : Subsystem
  PI Controller with Integral Anti-windup for HX6 : Subsystem
  P_demand (MW) PHX1 : Constant  Value=42
  P_demand (MW) PHX2 : Constant  Value=42
  P_demand (MW) PHX3 : Constant  Value=42
  Parasitic Heat Loss Resulting from DRACS HXs2 : Subsystem
  Primary Heat Exchanger Lumped Model #4 : Subsystem
  Primary Heat Exchanger Lumped Model #5 : Subsystem
  Primary Heat Exchanger Lumped Model #6 : Subsystem
  Ramp Power1 : Subsystem
  Ramp Power2 : Subsystem
  Ramp Power3 : Subsystem
  Reactor Outlet Temperature PI Controller1 : Subsystem
  Saturation3 : Saturate  UpperLimit=inf  LowerLimit=0
  Saturation4 : Saturate  UpperLimit=inf  LowerLimit=0
  Saturation5 : Saturate  UpperLimit=inf  LowerLimit=0
  Secondary-side RCP Dynamics #4 : Subsystem
  Secondary-side RCP Dynamics #5 : Subsystem
  Secondary-side RCP Dynamics #6 : Subsystem
  Sum2 : Sum  Inputs=|+-
  Sum5 : Sum  Inputs=|+-
  Secondary-Side HX massflow : Outport
  Secondary-Side HX Temp : Outport  Port=2
  wires:
  Reactor Outlet Temperature PI Controller1/1(Out1) -> Neutron Kinetics and Thermal Hydraulics/1(% Rod Withdrawn), Display31/1, Display34/1
  Parasitic Heat Loss Resulting from DRACS HXs2/3(Hot Leg Reduction) -> Sum5/2, Display17/1
  Parasitic Heat Loss Resulting from DRACS HXs2/1(Total Power Out) -> Display19/1
  Parasitic Heat Loss Resulting from DRACS HXs2/2(Power Lost) -> Display28/1
  Sum5/1 -> Display29/1, [HLtemp]
  Neutron Kinetics and Thermal Hydraulics/6(Thermal Power Extraction) -> Display32/1
  Neutron Kinetics and Thermal Hydraulics/5(Zonal Normalized Power) -> Display33/1
  Neutron Kinetics and Thermal Hydraulics/4(Normalized Power Out of Reactor) -> Display35/1
  Neutron Kinetics and Thermal Hydraulics/1(Lower Zone Rod Worth and Reactivity) -> Display20/1
  Neutron Kinetics and Thermal Hydraulics/2(Middle Zone Rod Worth and Reactivity) -> Display21/1
  Neutron Kinetics and Thermal Hydraulics/3(Upper Zone Rod Worth and Reactivity) -> Display25/1
  Sum2/1 -> Reactor Outlet Temperature PI Controller1/1(In1)
  Constant2/1 -> Sum2/1
  [m1] -> MATLAB Function/1(m1)
  [m2] -> MATLAB Function/2(m2)
  [m3] -> MATLAB Function/3(m3)
  [T1] -> MATLAB Function/4(T1)
  [T2] -> MATLAB Function/5(T2)
  [T3] -> MATLAB Function/6(T3)
  MATLAB Function/2(SHX_temp) -> Secondary-Side HX Temp/1
  MATLAB Function/1(SHX_massflow) -> Secondary-Side HX massflow/1
  RX_SHX Return Temp/1 -> [T_SHXreturn]
  [C1] -> Downcomer mixing dynamics/1(PHX Primary Flow 1)
  [C2] -> Downcomer mixing dynamics/2(PHX Primary Flow 2)
  [C3] -> Downcomer mixing dynamics/3(PHX Primary Flow 3)
  [D1] -> Downcomer mixing dynamics/4(PHX Primary Temp 1)
  [D2] -> Downcomer mixing dynamics/5(PHX Primary Temp 2)
  [D3] -> Downcomer mixing dynamics/6(PHX Primary Temp 3)
  Hot leg flow kg/s3/1 -> Primary Heat Exchanger Lumped Model #4/1(Primary mass flow  in), [C1]
  Hot leg flow kg/s4/1 -> [C2], Primary Heat Exchanger Lumped Model #5/1(Primary mass flow  in)
  Hot leg flow kg/s5/1 -> [C3], Primary Heat Exchanger Lumped Model #6/1(Primary mass flow  in)
  Primary Heat Exchanger Lumped Model #5/3(PHx1_HXout) -> Saturation5/1
  [HLtemp] -> Primary Heat Exchanger Lumped Model #4/2(Primary temp in)
  [HLtemp] -> Primary Heat Exchanger Lumped Model #5/2(Primary temp in)
  [HLtemp] -> Primary Heat Exchanger Lumped Model #6/2(Primary temp in)
  Primary Heat Exchanger Lumped Model #4/3(PHx1_HXout) -> Saturation4/1
  Primary Heat Exchanger Lumped Model #6/3(PHx1_HXout) -> Saturation3/1
  Saturation3/1 -> PI Controller with Integral Anti-windup for HX6/1(HX Power Produced), Display24/1
  Saturation4/1 -> PI Controller with Integral Anti-windup for HX4/1(HX Power Produced), Display22/1
  Ramp Power1/1(Current Demand) -> PI Controller with Integral Anti-windup for HX4/2(Power Setpoint)
  Ramp Power2/1(Current Demand) -> PI Controller with Integral Anti-windup for HX5/2(Power Setpoint)
  Ramp Power3/1(Current Demand) -> PI Controller with Integral Anti-windup for HX6/2(Power Setpoint)
  PI Controller with Integral Anti-windup for HX4/1(Control Action) -> Secondary-side RCP Dynamics #4/1(In1)
  Secondary-side RCP Dynamics #4/1(Out1) -> [m1], Primary Heat Exchanger Lumped Model #4/4(Secondary mass flow in)
  PI Controller with Integral Anti-windup for HX5/1(Control Action) -> Secondary-side RCP Dynamics #5/1(In1)
  Secondary-side RCP Dynamics #5/1(Out1) -> [m2], Primary Heat Exchanger Lumped Model #5/4(Secondary mass flow in)
  PI Controller with Integral Anti-windup for HX6/1(Control Action) -> Secondary-side RCP Dynamics #6/1(In1)
  Secondary-side RCP Dynamics #6/1(Out1) -> [m3], Primary Heat Exchanger Lumped Model #6/4(Secondary mass flow in), Display23/1
  Saturation5/1 -> PI Controller with Integral Anti-windup for HX5/1(HX Power Produced)
  [T_SHXreturn] -> Primary Heat Exchanger Lumped Model #4/3(Secondary temp in)
  [T_SHXreturn] -> Primary Heat Exchanger Lumped Model #5/3(Secondary temp in)
  [T_SHXreturn] -> Primary Heat Exchanger Lumped Model #6/3(Secondary temp in)
  Primary Heat Exchanger Lumped Model #4/1(PHx1_Tho) -> [D1]
  Primary Heat Exchanger Lumped Model #4/2(PHx1_Tco) -> [T1]
  Primary Heat Exchanger Lumped Model #5/2(PHx1_Tco) -> [T2]
  Primary Heat Exchanger Lumped Model #5/1(PHx1_Tho) -> [D2]
  Primary Heat Exchanger Lumped Model #6/2(PHx1_Tco) -> [T3]
  Primary Heat Exchanger Lumped Model #6/1(PHx1_Tho) -> [D3]
  Downcomer mixing dynamics/1(Primary Mass Flow Rate) -> [mdot_pri]
  [mdot_pri] -> Parasitic Heat Loss Resulting from DRACS HXs2/3(Primary Mass Flow Rate)
  [mdot_pri] -> Neutron Kinetics and Thermal Hydraulics/2(Primary Mass Flowrate)
  Downcomer mixing dynamics/2(Temperature to Reactor T-H) -> [T_cool_in]
  [T_cool_in] -> Parasitic Heat Loss Resulting from DRACS HXs2/2(T_cold)
  [T_cool_in] -> Neutron Kinetics and Thermal Hydraulics/3(Primary Coolant Temperature In)
  Neutron Kinetics and Thermal Hydraulics/7(T_hot) -> Display26/1, [T_react_out]
  [T_react_out] -> Parasitic Heat Loss Resulting from DRACS HXs2/1("T_hot ")
  [T_react_out] -> Sum5/1
  [T_react_out] -> Sum2/2
  P_demand (MW) PHX1/1 -> Ramp Power1/1(Max Demand)
  P_demand (MW) PHX2/1 -> Ramp Power2/1(Max Demand)
  P_demand (MW) PHX3/1 -> Ramp Power3/1(Max Demand)

== system SpatialKineticsOffline/RX #1/Downcomer mixing dynamics ==
  PHX Primary Flow 1 : Inport
  PHX Primary Flow 2 : Inport  Port=2
  PHX Primary Flow 3 : Inport  Port=3
  PHX Primary Temp 1 : Inport  Port=4
  PHX Primary Temp 2 : Inport  Port=5
  PHX Primary Temp 3 : Inport  Port=6
  Constant5 : Constant  Value=[0,downcomerTimeConstant]
  Display : Display
  Integrator : Integrator  InitialCondition=downIO
  MATLAB Function1 : MATLAB Function  TreatAsAtomicUnit=on
  Primary Mass Flow Rate : Outport
  Temperature to Reactor T-H : Outport  Port=2
  wires:
  PHX Primary Flow 1/1 -> MATLAB Function1/1(m1)
  PHX Primary Flow 2/1 -> MATLAB Function1/2(m2)
  PHX Primary Flow 3/1 -> MATLAB Function1/3(m3)
  PHX Primary Temp 1/1 -> MATLAB Function1/4(t1)
  PHX Primary Temp 2/1 -> MATLAB Function1/5(t2)
  PHX Primary Temp 3/1 -> MATLAB Function1/6(t3)
  MATLAB Function1/3(xdot) -> Integrator/1
  MATLAB Function1/1(y) -> Temperature to Reactor T-H/1
  Constant5/1 -> MATLAB Function1/7(constants)
  MATLAB Function1/2(mtotal) -> Primary Mass Flow Rate/1
  Integrator/1 -> MATLAB Function1/8(x), Display/1

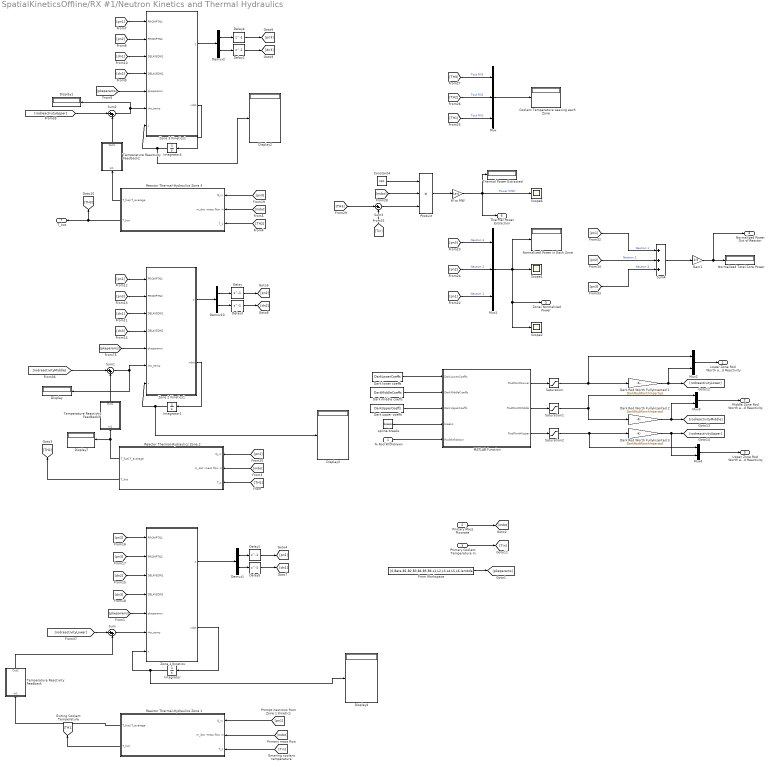
== system SpatialKineticsOffline/RX #1/Neutron Kinetics and Thermal Hydraulics ==
  % Rod Withdrawn : Inport
  Primary Mass Flowrate : Inport  Port=2
  Primary Coolant Temperature In : Inport  Port=3
  Constant4 : Constant  Value=cpc
  Coolant Temperature Leaving each Zone : Display
  Dark Rod Worth FullyInserted 1 : Gain  Gain=DarkRodWorthInserted
  Dark Rod Worth FullyInserted 2 : Gain  Gain=DarkRodWorthInserted
  Dark Rod Worth FullyInserted 3 : Gain  Gain=DarkRodWorthInserted
  Dark lower coeffs : Constant  Value=DarkLowerCoeffs
  Dark middle coeffs : Constant  Value=DarkMiddleCoeffs
  Dark upper coeffs : Constant  Value=DarkUpperCoeffs
  Delay{,1..5} (6 alike) : Delay  DelayLength=1  InitialCondition=0
  Demux1 : Demux  Outputs=2
  Demux10 : Demux  Outputs=2
  Demux2 : Demux  Outputs=2
  Display{,1..4,7} (6 alike) : Display
  From Workspace : FromWorkspace  VariableName=[0,Beta,B1,B2,B3,B4,B5,B6,L1,L2,L3,L4,L5,L6,lambda]  SampleTime=0
  Gain1 : Gain  Gain=1/3
  Integrator : Integrator  InitialCondition=zone1_IO
  Integrator1 : Integrator  InitialCondition=zone2_IO
  Integrator4 : Integrator  InitialCondition=zone3_IO
  MATLAB Function : MATLAB Function  TreatAsAtomicUnit=on
  Mux : Mux  Inputs=3
  Mux1 : Mux  Inputs=3
  Mux2 : Mux  Inputs=2
  Mux3 : Mux  Inputs=2
  Mux4 : Mux  Inputs=2
  Normalized Power in Each Zone : Display
  Normalized Total Core Power : Display
  Product : Product  Inputs=3
  Reactor Thermal-Hydraulics Zone 1 : Subsystem
  Reactor Thermal-Hydraulics Zone 2 : Subsystem
  Reactor Thermal-Hydraulics Zone 3 : Subsystem
  Saturation : Saturate  UpperLimit=inf  LowerLimit=0
  Saturation1 : Saturate  UpperLimit=inf  LowerLimit=0
  Saturation2 : Saturate  UpperLimit=inf  LowerLimit=0
  Scope1 : Scope
      settings: SaveName=ScopeData10
  Scope2 : Scope
      settings: SaveName=ScopeData11
  Scope6 : Scope
      settings: SaveName=ScopeData7
  Sum : Sum  Inputs=|++
  Sum1 : Sum  Inputs=|++
  Sum2 : Sum  Inputs=|++
  Sum3 : Sum  Inputs=|+-
  Sum4 : Sum  Inputs=+++
  Temperature Reactivity Feedback : Subsystem
  Temperature Reactivity Feedback2 : Subsystem
  Temperature Reactivity Feedback3 : Subsystem
  Thermal Power Extracted : Display
  W to MW : Gain  Gain=1e-6
  Zone 1 Kinetics : MATLAB Function  TreatAsAtomicUnit=on
  Zone 2 Kinetics1 : MATLAB Function  TreatAsAtomicUnit=on
  Zone 3 Kinetics1 : MATLAB Function  TreatAsAtomicUnit=on
  spline breaks : Constant  Value=breaks
  Lower Zone Rod Worth and Reactivity : Outport
  Middle Zone Rod Worth and Reactivity : Outport  Port=2
  Upper Zone Rod Worth and Reactivity : Outport  Port=3
  Normalized Power Out of Reactor : Outport  Port=4
  Zonal Normalized Power : Outport  Port=5
  Thermal Power Extraction : Outport  Port=6
  T_hot : Outport  Port=7
  wires:
  [pkeparams] -> Zone 2 Kinetics1/5(pkeparams)
  Demux1/2 -> Delay5/1
  From Workspace/1 -> [pkeparams]
  Reactor Thermal-Hydraulics Zone 2/1(T_fuel,T_average) -> Display7/1, Temperature Reactivity Feedback3/1(In1)
  [TH1] -> Reactor Thermal-Hydraulics Zone 2/3(T_c)
  Temperature Reactivity Feedback3/1(Out1) -> Sum1/2
  [pkeparams] -> Zone 1 Kinetics/5(pkeparams)
  Zone 1 Kinetics/1(y) -> Demux1/1
  Reactor Thermal-Hydraulics Zone 1/1(T_fuel,T_average) -> Temperature Reactivity Feedback/1(In1)
  Temperature Reactivity Feedback/1(Out1) -> Sum/2
  Demux1/1 -> Delay1/1
  Sum/1 -> Zone 1 Kinetics/6(rho_temp)
  [rodreactivityLower] -> Sum/1
  Sum1/1 -> Zone 2 Kinetics1/6(rho_temp), Display/1
  [rodreactivityMiddle] -> Sum1/1
  Mux/1 -> Coolant Temperature Leaving each Zone/1
  Reactor Thermal-Hydraulics Zone 1/2(T_hot) -> [TH1]
  [mdot] -> Reactor Thermal-Hydraulics Zone 2/2(m_dot -mass flow in)
  [mdot] -> Reactor Thermal-Hydraulics Zone 1/2(m_dot -mass flow in)
  Reactor Thermal-Hydraulics Zone 3/1(T_fuel,T_average) -> Temperature Reactivity Feedback2/1(In1)
  [TH2] -> Reactor Thermal-Hydraulics Zone 3/3(T_c)
  Reactor Thermal-Hydraulics Zone 3/2(T_hot) -> T_hot/1, [TH3]
  Temperature Reactivity Feedback2/1(Out1) -> Sum2/2
  Demux2/1 -> Delay4/1
  Sum2/1 -> Zone 3 Kinetics1/6(rho_temp), Display1/1
  [mdot] -> Reactor Thermal-Hydraulics Zone 3/2(m_dot -mass flow in)
  Delay5/1 -> [dn1]
  Demux2/2 -> Delay2/1
  Reactor Thermal-Hydraulics Zone 2/2(T_hot) -> [TH2]
  Demux10/1 -> Delay/1
  Demux10/2 -> Delay3/1
  Delay4/1 -> [pn3]
  Delay/1 -> [pn2]
  Delay1/1 -> [pn1]
  Delay3/1 -> [dn2]
  Delay2/1 -> [dn3]
  [rodreactivityUpper] -> Sum2/1
  [pn1] -> Zone 2 Kinetics1/1(PROMPTN1)
  [pn3] -> Zone 2 Kinetics1/2(PROMPTN2)
  [dn3] -> Zone 2 Kinetics1/4(DELAYEDN2)
  [dn1] -> Zone 2 Kinetics1/3(DELAYEDN1)
  [pn2] -> Zone 1 Kinetics/1(PROMPTN1)
  [pn3] -> Zone 1 Kinetics/2(PROMPTN2)
  [dn2] -> Zone 1 Kinetics/3(DELAYEDN1)
  [dn3] -> Zone 1 Kinetics/4(DELAYEDN2)
  [pn3] -> Reactor Thermal-Hydraulics Zone 3/1(Q_rx)
  [pn2] -> Reactor Thermal-Hydraulics Zone 2/1(Q_rx)
  [pn1] -> Reactor Thermal-Hydraulics Zone 1/1(Q_rx)
  Mux1/1 -> Scope1/1, Scope2/1, Zonal Normalized Power/1, Normalized Power in Each Zone/1
  [pn1] -> Mux1/3  "Neutron 1"
  [pn3] -> Mux1/1  "Neutron 3"
  [pn2] -> Mux1/2  "Neutron 2"
  [TH1] -> Mux/3  "Tout RX1"
  [TH2] -> Mux/2  "Tout RX2"
  [TH3] -> Mux/1  "Tout RX3"
  Constant4/1 -> Product/1
  [mdot] -> Product/2
  Sum3/1 -> Product/3
  [TH3] -> Sum3/1
  [Tin] -> Reactor Thermal-Hydraulics Zone 1/3(T_c)
  [Tin] -> Sum3/2
  Product/1 -> W to MW/1
  W to MW/1 -> Scope6/1, Thermal Power Extraction/1, Thermal Power Extracted/1  "Power (MW)"
  [pn1] -> Sum4/1  "Neutron 1"
  [pn3] -> Sum4/3  "Neutron 3"
  [pn2] -> Sum4/2  "Neutron 2"
  Sum4/1 -> Gain1/1
  Gain1/1 -> Normalized Power Out of Reactor/1, Normalized Total Core Power/1
  spline breaks/1 -> MATLAB Function/4(breaks)
  Dark upper coeffs/1 -> MATLAB Function/3(DarkUpperCoeffs)
  Dark middle coeffs/1 -> MATLAB Function/2(DarkMiddleCoeffs)
  Dark lower coeffs/1 -> MATLAB Function/1(DarkLowerCoeffs)
  MATLAB Function/1(RodWorthLower) -> Saturation/1
  MATLAB Function/2(RodWorthMiddle) -> Saturation1/1
  MATLAB Function/3(RodWorthUpper) -> Saturation2/1
  % Rod Withdrawn/1 -> MATLAB Function/5(RodWithdrawn)
  Saturation/1 -> Mux2/1, Dark Rod Worth FullyInserted 1/1
  Saturation1/1 -> Dark Rod Worth FullyInserted 2/1, Mux3/1
  Saturation2/1 -> Mux4/1, Dark Rod Worth FullyInserted 3/1
  Dark Rod Worth FullyInserted 1/1 -> Mux2/2, [rodreactivityLower]
  Dark Rod Worth FullyInserted 2/1 -> Mux3/2, [rodreactivityMiddle]
  Dark Rod Worth FullyInserted 3/1 -> Mux4/2, [rodreactivityUpper]
  Primary Mass Flowrate/1 -> [mdot]
  Primary Coolant Temperature In/1 -> [Tin]
  Mux2/1 -> Lower Zone Rod Worth and Reactivity/1
  Mux3/1 -> Middle Zone Rod Worth and Reactivity/1
  Mux4/1 -> Upper Zone Rod Worth and Reactivity/1
  Integrator4/1 -> Zone 3 Kinetics1/7(x), Display2/1
  Zone 3 Kinetics1/2(xdot) -> Integrator4/1
  [pkeparams] -> Zone 3 Kinetics1/5(pkeparams)
  [dn2] -> Zone 3 Kinetics1/4(DELAYEDN2)
  [dn1] -> Zone 3 Kinetics1/3(DELAYEDN1)
  [pn2] -> Zone 3 Kinetics1/2(PROMPTN2)
  [pn1] -> Zone 3 Kinetics1/1(PROMPTN1)
  Zone 3 Kinetics1/1(y) -> Demux2/1
  Zone 2 Kinetics1/2(xdot) -> Integrator1/1
  Integrator1/1 -> Display3/1, Zone 2 Kinetics1/7(x)
  Zone 2 Kinetics1/1(y) -> Demux10/1
  Zone 1 Kinetics/2(xdot) -> Integrator/1
  Integrator/1 -> Display4/1, Zone 1 Kinetics/7(x)

== system SpatialKineticsOffline/RX #1/PI Controller with Integral Anti-windup for HX1 ==
  HX Power Produced : Inport
  Power Setpoint : Inport  Port=2
  Anti-windup gain : Gain  Gain=15
  Cold_massflow_high : Constant  Value=370
  Cold_massflow_low : Constant  Value=0
  Display{,1..3} (4 alike) : Display
  Integrator : Integrator  InitialCondition=PHX_PI_IO
  Ki : Gain  Gain=0.14145998
  Kp : Gain  Gain=1.083074
  Saturation Dynamic : simulink/Discontinuities/Saturation Dynamic  OutMin=[]  OutMax=[]  OutDataTypeStr=Inherit: Same as second input  OutDataType=fixdt(1, 16)  OutScaling=2^-10  DoSatur=off
  Scope : Scope
      settings: YMin=20  YMax=42
  Sum12 : Sum  Inputs=+-|
  Sum13 : Sum  Inputs=|+-
  Sum14 : Sum  Inputs=|+-
  Sum15 : Sum  Inputs=|++
  Control Action : Outport
  tag scope: PHX1_control=global, PHX1_error=global
  wires:
  HX Power Produced/1 -> Sum14/2
  Cold_massflow_low/1 -> Saturation Dynamic/3
  Cold_massflow_high/1 -> Saturation Dynamic/1
  Sum14/1 -> [PHX1_error], Scope/1, Display/1, Kp/1, Sum13/1
  Power Setpoint/1 -> Sum14/1
  Sum12/1 -> Anti-windup gain/1
  Integrator/1 -> Display3/1, Sum15/2
  Anti-windup gain/1 -> Sum13/2
  Sum13/1 -> Ki/1
  Ki/1 -> Integrator/1
  Kp/1 -> Sum15/1
  Saturation Dynamic/1 -> [PHX1_control], Display1/1, Sum12/2, Control Action/1
  Sum15/1 -> Sum12/1, Display2/1, Saturation Dynamic/2
